simulink model "controlValidation"  (R2021a)
settings: Solver=VariableStepAuto  StartTime=0.0  StopTime=10.0  RelTol=1e-3
libraries: pid_lib x1
settings Model: Creator=filip  LastModifiedBy=filip

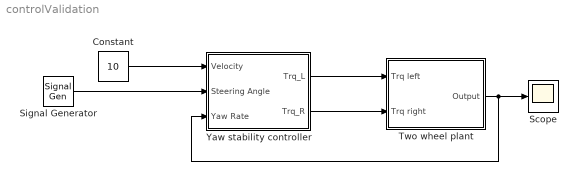
== system controlValidation ==
  Constant : Constant  Value=10
  Scope : Scope
  Signal Generator : SignalGenerator  Amplitude=2  Units=rad/sec
  Two wheel plant : Subsystem
  Yaw stability controller : Subsystem
  wires:
  Constant/1 -> Yaw stability controller/1(Velocity)
  Signal Generator/1 -> Yaw stability controller/2(Steering Angle)
  Two wheel plant/1(Output) -> Yaw stability controller/3(Yaw Rate), Scope/1
  Yaw stability controller/2(Trq_R) -> Two wheel plant/2(Trq right)
  Yaw stability controller/1(Trq_L) -> Two wheel plant/1(Trq left)

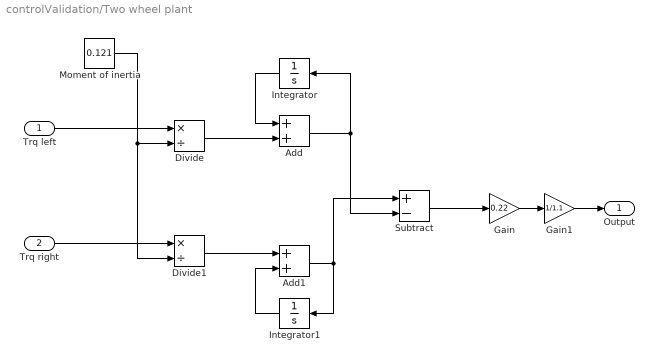
== system controlValidation/Two wheel plant ==
  Trq left : Inport
  Trq right : Inport  Port=2
  Add : Sum
  Add1 : Sum
  Divide : Product  Inputs=*/
  Divide1 : Product  Inputs=*/
  Gain : Gain  Gain=0.22
  Gain1 : Gain  Gain=1/1.1
  Integrator : Integrator
  Integrator1 : Integrator
  Moment of inertia : Constant  Value=0.121
  Subtract : Sum  Inputs=+-
  Output : Outport
  wires:
  Trq left/1 -> Divide/1
  Trq right/1 -> Divide1/1
  Moment of inertia/1 -> Divide1/2, Divide/2
  Divide1/1 -> Add1/1
  Divide/1 -> Add/2
  Add/1 -> Subtract/2, Integrator/1
  Integrator/1 -> Add/1
  Add1/1 -> Integrator1/1, Subtract/1
  Integrator1/1 -> Add1/2
  Subtract/1 -> Gain/1
  Gain/1 -> Gain1/1
  Gain1/1 -> Output/1

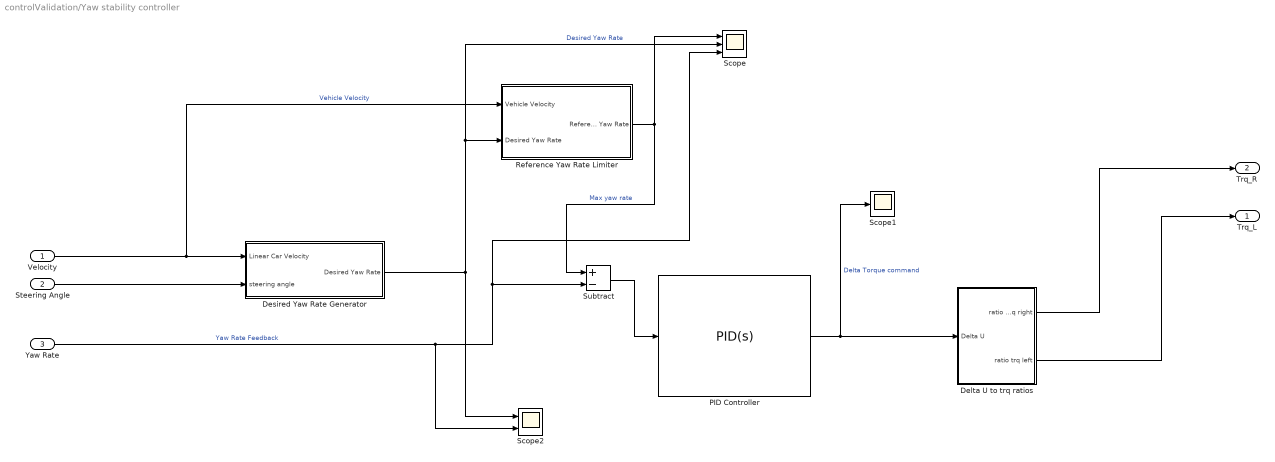
== system controlValidation/Yaw stability controller ==
  Velocity : Inport  ClipboardFcn=set_param(gcb,'BackgroundColor','red');
  Steering Angle : Inport  Port=2
  Yaw Rate : Inport  Port=3
  Delta U to trq ratios : Subsystem
  Desired Yaw Rate Generator : Subsystem
  "PID Controller " : pid_lib/PID Controller  Controller=PID  Form=Parallel  TimeDomain=Continuous-time  UseExternalTs=off  SampleTime=-1  IntegratorMethod=Forward Euler  FilterMethod=Forward Euler  ControllerParametersSource=internal  P=0  I=47.6665576023681  D=0  UseFilter=on  N=100  TunerSelectOption=Transfer Function Based (PID Tuner App)  InitialConditionSource=internal  InitialConditionForIntegrator=0  InitialConditionForFilter=0  DifferentiatorICPrevScaledInput=0  ExternalReset=none  TrackingMode=off  Kt=1  LimitOutput=off  SatLimitsSource=internal  UpperSaturationLimit=240  LowerSaturationLimit=0  LinearizeAsGain=off  AntiWindupMode=clamping  Kb=1  POutMin=[]  POutMax=[]  IOutMin=[]  IOutMax=[]  DOutMin=[]  DOutMax=[]  NOutMin=[]  NOutMax=[]  SumOutMin=[]  SumOutMax=[]  SaturationOutMin=[]  SaturationOutMax=[]  PParamMin=[]  PParamMax=[]  IParamMin=[]  IParamMax=[]  DParamMin=[]  DParamMax=[]  NParamMin=[]  NParamMax=[]  KbParamMin=[]  KbParamMax=[]  KtParamMin=[]  KtParamMax=[]  KbOutMin=[]  KbOutMax=[]  KtOutMin=[]  KtOutMax=[]  IntegratorOutMin=[]  IntegratorOutMax=[]  FilterOutMin=[]  FilterOutMax=[]  SumI1OutMin=[]  SumI1OutMax=[]  SumI2OutMin=[]  SumI2OutMax=[]  SumI3OutMin=[]  SumI3OutMax=[]  SumI4OutMin=[]  SumI4OutMax=[]  SumDOutMin=[]  SumDOutMax=[]  DifferentiatorOutMin=[]  DifferentiatorOutMax=[]  FilterDiffOutCoefMin=[]  FilterDiffOutCoefMax=[]  ReciprocalOutMin=[]  ReciprocalOutMax=[]  SumDenOutMin=[]  SumDenOutMax=[]  SumNumOutMin=[]  SumNumOutMax=[]  DivideOutMin=[]  DivideOutMax=[]  UdiffTsProdOutMin=[]  UdiffTsProdOutMax=[]  NTsProdOutMin=[]  NTsProdOutMax=[]  UintegralTsProdOutMin=[]  UintegralTsProdOutMax=[]  UngainTsProdOutMin=[]  UngainTsProdOutMax=[]  IntegratorContinuousStateAttributes=''  IntegratorStateMustResolveToSignalObject=off  IntegratorRTWStateStorageClass=Auto  FilterContinuousStateAttributes=''  FilterStateMustResolveToSignalObject=off  FilterRTWStateStorageClass=Auto  ParallelPVariant=InternalParameters  IdealPVariant=Disabled  IVariant=InternalParameters  DVariant=InternalParameters  IntegratorVariant=Continuous  SatVariant=Disabled  AWVariant=Passthrough  PCopyVariant=Disabled  TRVariant=Disabled  FdbkBlocksVariant=Forward  IdealPFdbkVariant=Disabled  SatFdbkVariant=Disabled  DerivativeFilterVariant=ContFilter  NVariant=InternalParameters  NCopyVariant=Disabled  FilterICVariant=InternalICsFilter  IntegratorICVariant=InternalICs  ExternalResetVariant=Disabled  TRSumVariant=Passthrough  SumFdbkVariant=Disabled  SumVariant=Sum_PID  TsampFilterVariant=InternalTs  TsampNgainVariant=Passthrough  TsampIntegralVariant=Passthrough  ExternalSaturationOutDataTypeStr=Inherit: Same as second input
  Reference Yaw Rate Limiter : Subsystem
  Scope : Scope  NumInputPorts=3
  Scope1 : Scope
  Scope2 : Scope  NumInputPorts=2
  Subtract : Sum  Inputs=+-
  Trq_L : Outport
  Trq_R : Outport  Port=2
  wires:
  "PID Controller "/1 -> Scope1/1, Delta U to trq ratios/1(Delta U)  "Delta Torque command"
  Desired Yaw Rate Generator/1(Desired Yaw Rate) -> Scope2/1, Reference Yaw Rate Limiter/2(Desired Yaw Rate), Scope/2  "Desired Yaw Rate"
  Subtract/1 -> "PID Controller "/1
  Yaw Rate/1 -> Scope2/2, Subtract/2, Scope/3  "Yaw Rate Feedback"
  Velocity/1 -> Desired Yaw Rate Generator/1(Linear Car Velocity), Reference Yaw Rate Limiter/1(Vehicle Velocity)  "Vehicle Velocity"
  Steering Angle/1 -> Desired Yaw Rate Generator/2(steering angle)
  Reference Yaw Rate Limiter/1(Reference Yaw Rate) -> Subtract/1, Scope/1  "Max yaw rate"
  Delta U to trq ratios/1(" ratio trq right") -> Trq_R/1
  Delta U to trq ratios/2(ratio trq left) -> Trq_L/1

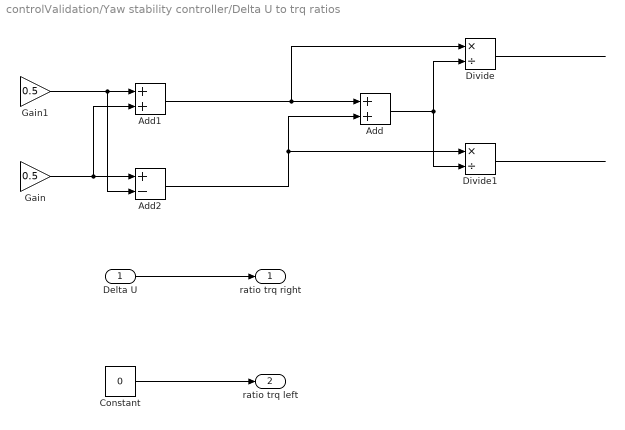
== system controlValidation/Yaw stability controller/Delta U to trq ratios ==
  Delta U : Inport
  Add : Sum
  Add1 : Sum
  Add2 : Sum  Inputs=+-
  Constant : Constant  Value=0
  Divide : Product  Inputs=*/
  Divide1 : Product  Inputs=*/
  Gain : Gain  Gain=0.5
  Gain1 : Gain  Gain=0.5
  " ratio trq right" : Outport
  ratio trq left : Outport  Port=2
  wires:
  Delta U/1 -> " ratio trq right"/1
  Constant/1 -> ratio trq left/1
  Gain1/1 -> Add2/2, Add1/1
  ? -> Gain/1
  Divide1/1 -> ?
  Gain/1 -> Add2/1, Add1/2
  ? -> Gain1/1
  Add1/1 -> Divide/1, Add/1
  Add2/1 -> Divide1/1, Add/2
  Add/1 -> Divide/2, Divide1/2
  Divide/1 -> ?

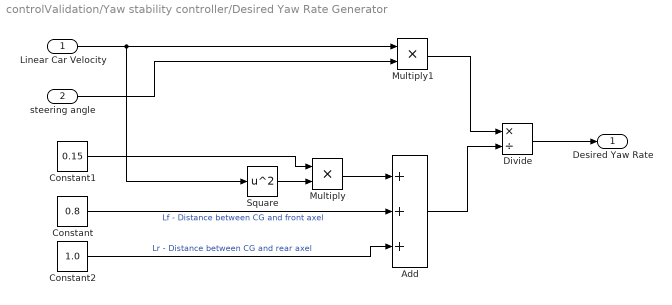
== system controlValidation/Yaw stability controller/Desired Yaw Rate Generator ==
  Linear Car Velocity : Inport
  steering angle : Inport  Port=2
  Add : Sum  Inputs=+++
  Constant : Constant  Value=0.8
  Constant1 : Constant  Value=0.15
  Constant2 : Constant  Value=1.0
  Divide : Product  Inputs=*/
  Multiply : Product
  Multiply1 : Product
  Square : Math  Operator=square  SignedPower=on  SaturateOnIntegerOverflow=on
  Desired Yaw Rate : Outport  VectorParamsAs1DForOutWhenUnconnected=off
  wires:
  Constant1/1 -> Multiply/1
  steering angle/1 -> Multiply1/2
  Divide/1 -> Desired Yaw Rate/1
  Linear Car Velocity/1 -> Square/1, Multiply1/1
  Multiply/1 -> Add/1
  Multiply1/1 -> Divide/1
  Square/1 -> Multiply/2
  Constant/1 -> Add/2  "Lf - Distance between CG and front axel"
  Constant2/1 -> Add/3  "Lr - Distance between CG and rear axel"
  Add/1 -> Divide/2

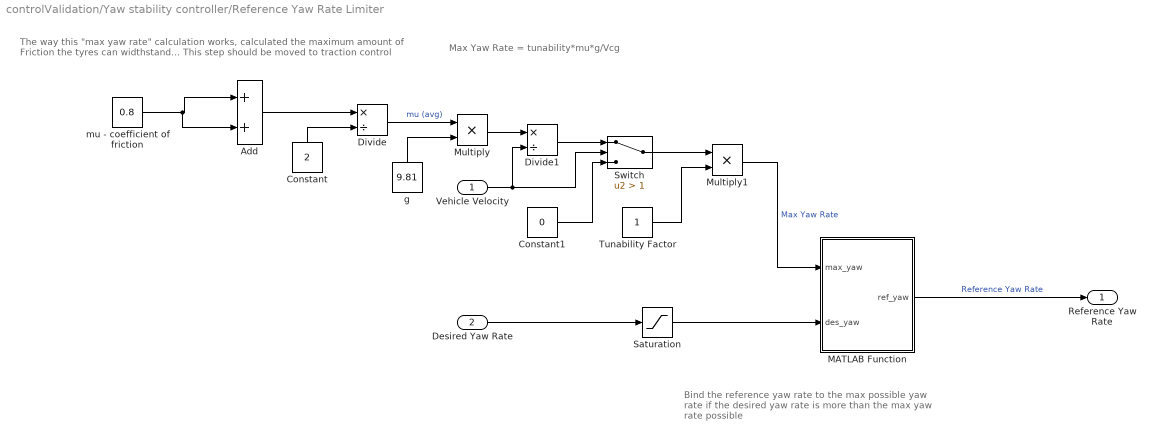
== system controlValidation/Yaw stability controller/Reference Yaw Rate Limiter ==
  note: Bind the reference yaw rate to the max possible yaw rate if the desired yaw rate is more than the max yaw rate possible
  note: Max Yaw Rate = tunability*mu*g/Vcg
  note: The way this "max yaw rate" calculation works, calculated the maximum amount of
      | Friction the tyres can widthstand... This step should be moved to traction control
  Vehicle Velocity : Inport
  Desired Yaw Rate : Inport  Port=2
  Add : Sum
  Constant : Constant  Value=2
  Constant1 : Constant  Value=0
  Divide : Product  Inputs=*/
  Divide1 : Product  Inputs=*/
  MATLAB Function : MATLAB Function  TreatAsAtomicUnit=on
  Multiply : Product
  Multiply1 : Product
  Saturation : Saturate  UpperLimit=10  LowerLimit=-10
  Switch : Switch  Criteria=u2 > Threshold  Threshold=1
  Tunability Factor : Constant
  g : Constant  Value=9.81
  mu - coefficient of friction : Constant  Value=0.8
  Reference Yaw Rate : Outport  VectorParamsAs1DForOutWhenUnconnected=off
  wires:
  Desired Yaw Rate/1 -> Saturation/1
  MATLAB Function/1(ref_yaw) -> Reference Yaw Rate/1  "Reference Yaw Rate"
  Add/1 -> Divide/1
  Constant/1 -> Divide/2
  Divide/1 -> Multiply/1  "mu (avg)"
  Multiply/1 -> Divide1/1
  Vehicle Velocity/1 -> Switch/2, Divide1/2
  g/1 -> Multiply/2
  Tunability Factor/1 -> Multiply1/2
  Multiply1/1 -> MATLAB Function/1(max_yaw)  "Max Yaw Rate"
  Divide1/1 -> Switch/1
  Constant1/1 -> Switch/3
  Switch/1 -> Multiply1/1
  Saturation/1 -> MATLAB Function/2(des_yaw)
  mu - coefficient of friction/1 -> Add/2, Add/1

== matlab function controlValidation/Yaw stability controller/Reference Yaw Rate Limiter/MATLAB Function ==
  data: max_yaw input; ref_yaw output; des_yaw input
function ref_yaw = fcn(max_yaw, des_yaw)
    if abs(des_yaw) > max_yaw
        if des_yaw >= 0
            ref_yaw = max_yaw;
        else
            ref_yaw = -max_yaw;
        end      
    else 
        ref_yaw = des_yaw;
    end
